simulink model "soal2_1"  (R2023b)
settings: Solver=ode4  StartTime=0.0  StopTime=30  FixedStep=0.01  RelTol=1e-3
InitFcn:
  | Ts = 0.01;
settings Model: Creator=amir  LastModifiedBy=amir

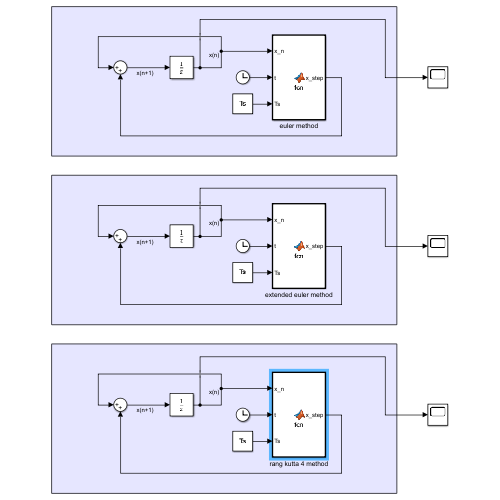
[thumbnail: Simulink's stored preview of the top-level diagram]
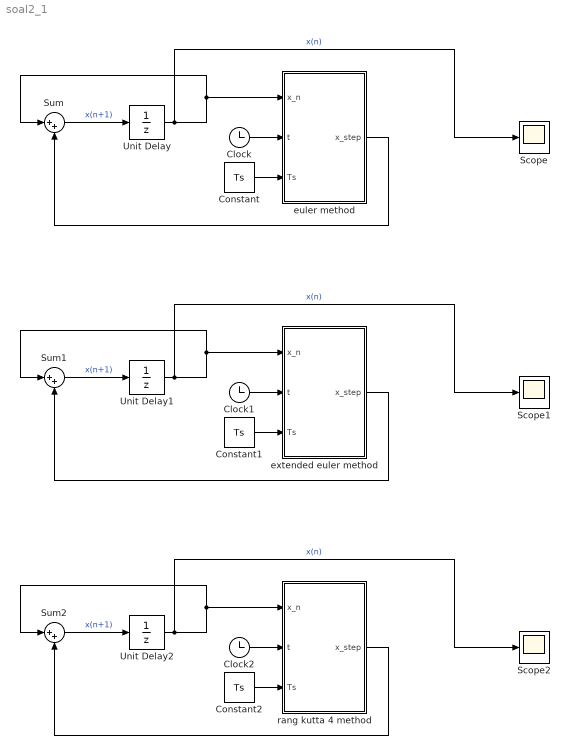
== system soal2_1 ==
  Clock : Clock
  Clock1 : Clock
  Clock2 : Clock
  Constant : Constant  Value=Ts
  Constant1 : Constant  Value=Ts
  Constant2 : Constant  Value=Ts
  Scope : Scope
  Scope1 : Scope
  Scope2 : Scope
  Sum : Sum  Inputs=|++
  Sum1 : Sum  Inputs=|++
  Sum2 : Sum  Inputs=|++
  Unit Delay : UnitDelay  SampleTime=-1  HasFrameUpgradeWarning=on
  Unit Delay1 : UnitDelay  SampleTime=-1  HasFrameUpgradeWarning=on
  Unit Delay2 : UnitDelay  SampleTime=-1  HasFrameUpgradeWarning=on
  euler method : MATLAB Function  TreatAsAtomicUnit=on
  extended euler method : MATLAB Function  TreatAsAtomicUnit=on
  rang kutta 4 method : MATLAB Function  TreatAsAtomicUnit=on
  wires:
  Sum/1 -> Unit Delay/1  "x(n+1)"
  Unit Delay/1 -> Scope/1, Sum/1, euler method/1(x_n)  "x(n)"
  Clock/1 -> euler method/2(t)
  Constant/1 -> euler method/3(Ts)
  euler method/1(x_step) -> Sum/2
  Unit Delay1/1 -> Scope1/1, Sum1/1, extended euler method/1(x_n)  "x(n)"
  Sum1/1 -> Unit Delay1/1  "x(n+1)"
  Clock1/1 -> extended euler method/2(t)
  extended euler method/1(x_step) -> Sum1/2
  Constant1/1 -> extended euler method/3(Ts)
  Constant2/1 -> rang kutta 4 method/3(Ts)
  Unit Delay2/1 -> Scope2/1, Sum2/1, rang kutta 4 method/1(x_n)  "x(n)"
  Sum2/1 -> Unit Delay2/1  "x(n+1)"
  Clock2/1 -> rang kutta 4 method/2(t)
  rang kutta 4 method/1(x_step) -> Sum2/2

== matlab function soal2_1/euler method ==
  data: x_n input; x_step output; t input; Ts input
function x_step = fcn(x_n, t, Ts)

x_step = (-7 * x_n + 0.1 * 2 * sin(4 * pi * t + pi/4) ) * Ts;

== matlab function soal2_1/rang kutta 4 method ==
  data: x_n input; x_step output; t input; Ts input
function x_step = fcn(x_n, t, Ts)

d_x1 = (-7 * x_n + 0.1 * 2 * sin(4 * pi * t + pi/4) ) * Ts;
d_x2 = (-7 * (x_n + d_x1/2) + 0.1 * 2 * sin(4 * pi * t + pi/4) ) * Ts;
d_x3 = (-7 * (x_n + d_x2/2) + 0.1 * 2 * sin(4 * pi * t + pi/4) ) * Ts;
d_x4 = (-7 * (x_n + d_x3) + 0.1 * 2 * sin(4 * pi * t + pi/4) ) * Ts;

x_step = (1/6) * (d_x1 + 2 * d_x2 + 2 * d_x3 + d_x4);

== matlab function soal2_1/extended euler method ==
  data: x_n input; x_step output; t input; Ts input
function x_step = fcn(x_n, t, Ts)

d_x1 = (-7 * x_n + 0.1 * 2 * sin(4 * pi * t + pi/4) ) * Ts;
d_x2 = (-7 * (x_n + d_x1) + 0.1 * 2 * sin(4 * pi * t + pi/4) ) * Ts;
x_step = 0.5 * (d_x1 + d_x2);
